simulink model "simulation01"  (R2024a)
settings: Solver=VariableStepAuto  StartTime=0.0  StopTime=50  RelTol=1e-3
values from neighbouring files (symbols this model uses):
  Ax = 0.3    [StateSpace.m]    (also in StateSpace00.m)
  Ay = 0.2    [StateSpace.m]    (also in StateSpace00.m)
  Az = 0.1    [StateSpace.m]    (also in StateSpace00.m)
  Cd = 0.4    [StateSpace.m]    (also in StateSpace00.m)
  g = 9.81    [StateSpace.m]    (also in StateSpace00.m = 9.8)
  Ix = (1/12) * m * (b^2 + c^2)    (= 0.416666666667)    [StateSpace.m]    (also in StateSpace00.m = 10)
  Iy = (1/12) * m * (a^2 + c^2)    (= 0.683333333333)    [StateSpace.m]    (also in StateSpace00.m = 20)
  Iz = (1/12) * m * (a^2 + b^2)    (= 0.566666666667)    [StateSpace.m]    (also in StateSpace00.m = 30)
  L = 5    [StateSpace.m]
  m = 5    [StateSpace.m]    (also in StateSpace00.m)
  rho = 1.225    [StateSpace.m]    (also in StateSpace00.m)
settings Model: Creator=swh  LastModifiedBy=swh
settings DebuggingCC: UnderSpecifiedDimensionMsg=warning

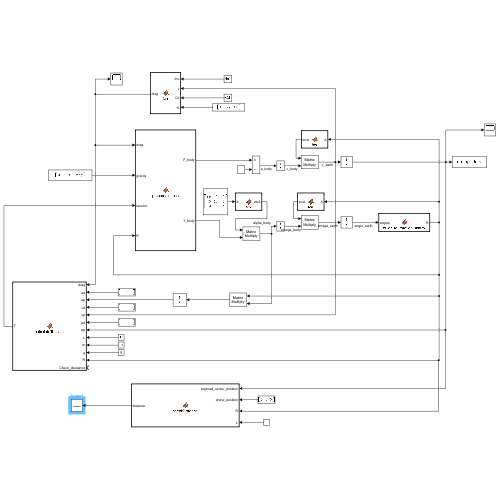
[thumbnail: Simulink's stored preview of the top-level diagram]
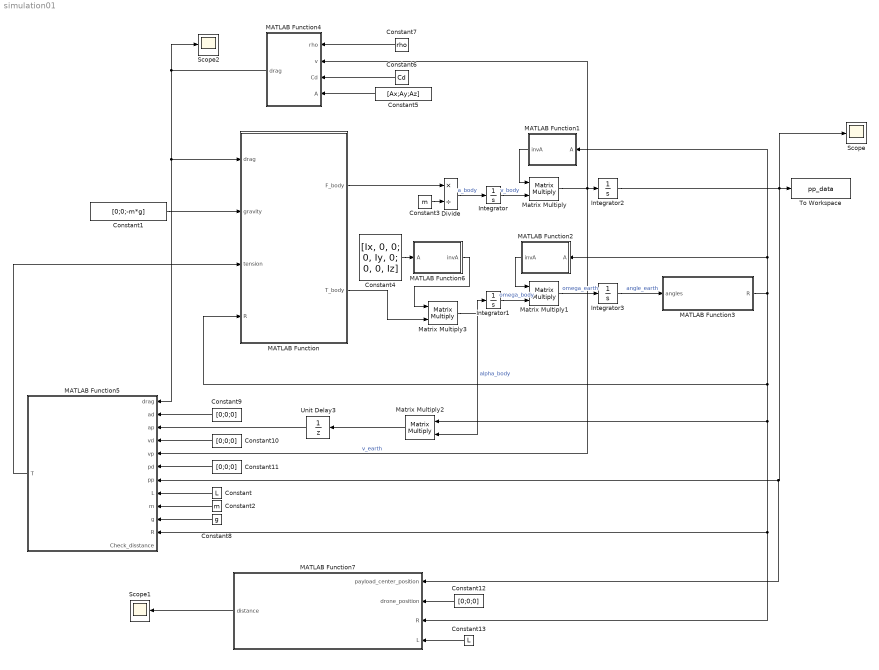
== system simulation01 ==
  Constant : Constant  Value=L
  Constant1 : Constant  Value=[0;0;-m*g]
  Constant{9..12} (4 alike) : Constant  Value=[0;0;0]
  Constant13 : Constant  Value=L
  Constant2 : Constant  Value=m
  Constant3 : Constant  Value=m
  Constant4 : Constant  Value=[Ix, 0, 0; 0, Iy, 0; 0, 0, Iz]
  Constant5 : Constant  Value=[Ax;Ay;Az]
  Constant6 : Constant  Value=Cd
  Constant7 : Constant  Value=rho
  Constant8 : Constant  Value=g
  Divide : Product  Inputs=*/
  Integrator : Integrator
  Integrator1 : Integrator
  Integrator2 : Integrator  InitialCondition=[0,-3,-4]
  Integrator3 : Integrator
  MATLAB Function : MATLAB Function  TreatAsAtomicUnit=on
  MATLAB Function1 : MATLAB Function  TreatAsAtomicUnit=on
  MATLAB Function2 : MATLAB Function  TreatAsAtomicUnit=on
  MATLAB Function3 : MATLAB Function  TreatAsAtomicUnit=on
  MATLAB Function4 : MATLAB Function  TreatAsAtomicUnit=on
  MATLAB Function5 : MATLAB Function  TreatAsAtomicUnit=on
  MATLAB Function6 : MATLAB Function  TreatAsAtomicUnit=on
  MATLAB Function7 : MATLAB Function  TreatAsAtomicUnit=on
  Matrix Multiply{,1..3} (4 alike) : Product  Multiplication=Matrix(*)
  Scope : Scope
  Scope1 : Scope
  Scope2 : Scope
  To Workspace : ToWorkspace  VariableName=pp_data  SaveFormat=Structure With Time  SampleTime=-1
  Unit Delay3 : UnitDelay  SampleTime=-1  HasFrameUpgradeWarning=on
  wires:
  Constant1/1 -> MATLAB Function/2(gravity)
  MATLAB Function/1(F_body) -> Divide/1
  Constant3/1 -> Divide/2
  MATLAB Function/2(T_body) -> Matrix Multiply3/2
  Divide/1 -> Integrator/1  "a_body"
  Matrix Multiply3/1 -> Matrix Multiply2/2, Integrator1/1  "alpha_body"
  Matrix Multiply/1 -> MATLAB Function4/2(v), MATLAB Function5/5(vp), Integrator2/1  "v_earth"
  Matrix Multiply1/1 -> Integrator3/1  "omega_earth"
  Integrator3/1 -> MATLAB Function3/1(angles)  "angle_earth"
  Constant5/1 -> MATLAB Function4/4(A)
  Constant6/1 -> MATLAB Function4/3(Cd)
  Constant7/1 -> MATLAB Function4/1(rho)
  Matrix Multiply2/1 -> Unit Delay3/1
  MATLAB Function4/1(drag) -> MATLAB Function/1(drag), MATLAB Function5/1(drag), Scope2/1
  Constant9/1 -> MATLAB Function5/2(ad)
  Constant10/1 -> MATLAB Function5/4(vd)
  Constant11/1 -> MATLAB Function5/6(pd)
  Constant/1 -> MATLAB Function5/8(L)
  Constant2/1 -> MATLAB Function5/9(m)
  Constant8/1 -> MATLAB Function5/10(g)
  MATLAB Function5/1(T) -> MATLAB Function/3(tension)
  Integrator/1 -> Matrix Multiply/2  "v_body"
  MATLAB Function1/1(invA) -> Matrix Multiply/1
  Integrator1/1 -> Matrix Multiply1/2  "omega_body"
  MATLAB Function2/1(invA) -> Matrix Multiply1/1
  Constant4/1 -> MATLAB Function6/1(A)
  MATLAB Function6/1(invA) -> Matrix Multiply3/1
  MATLAB Function3/1(R) -> MATLAB Function7/3(R), MATLAB Function5/11(R), Matrix Multiply2/1, MATLAB Function/4(R), MATLAB Function2/1(A), MATLAB Function1/1(A)
  Unit Delay3/1 -> MATLAB Function5/3(ap)
  Constant12/1 -> MATLAB Function7/2(drone_position)
  Constant13/1 -> MATLAB Function7/4(L)
  MATLAB Function7/1(distance) -> Scope1/1
  Integrator2/1 -> Scope/1, MATLAB Function7/1(payload_center_position), MATLAB Function5/7(pp), To Workspace/1

== matlab function simulation01/MATLAB Function1 ==
  data: A input; invA output
function invA = fcn(A)
% 计算矩阵 A 的逆
% 输入: A (3x3 矩阵)
% 输出: invA (A 的逆矩阵)
invA = inv(A);  % 使用 MATLAB 的 inv 函数
end

== matlab function simulation01/MATLAB Function ==
  data: drag input size=[3,1]; F_body output size=[3,1]; gravity input size=[3,1]; tension input size=[3,1]; R input size=[3,3]; T_body output size=[3,1]
function [F_body, T_body] = process_forces(drag, gravity, tension, R)
   
    c = 0.8; % The length of the rectangular prism along the z-axis
    r_top = [0;0;0.5 * c];
    % Convert forces from the Earth coordinate system to the body coordinate system
    drag_body = R * drag;
    gravity_body = R * gravity;
    tension_body = R * tension;
    
    % Calculate the resultant force in the body coordinate system
    F_body = drag_body + gravity_body + tension_body;
    
    % In this example, assume the torque is zero (this can be adjusted based on specific requirements)
    p_top = R * r_top;
    r = - p_top;
    T_body = cross(r, tension);  % Calculate the torque based on actual needs
    
end

== matlab function simulation01/MATLAB Function2 ==
  data: A input; invA output
function invA = fcn(A)
% 计算矩阵 A 的逆
% 输入: A (3x3 矩阵)
% 输出: invA (A 的逆矩阵)
invA = inv(A);  % 使用 MATLAB 的 inv 函数
end

== matlab function simulation01/MATLAB Function3 ==
  data: angles input; R output
function R = euler_to_rotation_matrix(angles)
% Calculate the rotation matrix for the given Euler angles
% Input: angles (3x1 column vector) containing Euler angles [phi; theta; psi]
% Output: R (3x3 rotation matrix)

% Extract Euler angles
phi = angles(1);   % Angle around the x-axis
theta = angles(2); % Angle around the y-axis
psi = angles(3);   % Angle around the z-axis

% Rotation matrix around the x-axis
Rx = [1, 0, 0;
      0, cos(phi), -sin(phi);
      0, sin(phi), cos(phi)];

% Rotation matrix around the y-axis
Ry = [cos(theta), 0, sin(theta);
      0, 1, 0;
      -sin(theta), 0, cos(theta)];

% Rotation matrix around the z-axis
Rz = [cos(psi), -sin(psi), 0;
      sin(psi), cos(psi), 0;
      0, 0, 1];

% Calculate the final rotation matrix
R = Rz * Ry * Rx;
end

== matlab function simulation01/MATLAB Function4 ==
  data: rho input; drag output size=[3,1]; v input size=[3,1]; Cd input; A input
function drag = fcn(rho, v, Cd, A)
    % 计算速度的大小
    speed = sqrt(v(1)^2 + v(2)^2 + v(3)^2);
    
    % 计算速度方向向量（单位向量）
    if speed ~= 0
        unit_v = v / speed;
    else
        % 如果速度为零，单位向量也为零
        unit_v = [0; 0; 0];
    end
    
    % 计算拖拽力的大小
    drag_magnitude = 0.5 * rho * speed^2 * Cd * A;
    
    % 计算拖拽力的方向和大小
    drag = -drag_magnitude .* unit_v; % 按元素相乘

end

== matlab function simulation01/MATLAB Function5 ==
  data: drag input; ad input; T output size=[3,1]; ap input; vd input; vp input; pd input; pp input; L input; m input; g input; R input; Check_disstance input
function T = calculateTension(drag, ad, ap, vd, vp, pd, pp, L, m, g, R, Check_disstance)
% Calculate the components of the rope tension in the x, y, and z directions for a 3D pendulum
%
% Inputs:
%   ad, ap - Acceleration components of the object at two different points
%   vd, vp - Velocity components of the object at two different points
%   pd, pp - Coordinates of the suspension point and the object
%   L - Length of the rope
%   m - Mass of the object
%   g - Acceleration due to gravity
%
% Output:
%   T - Tension components in the x, y, and z directions, in the form [Tx; Ty; Tz]

% Calculate displacement vector
c = 0.8;
r_top = [0;0;0.5 * c];
p_top = R * r_top;
p_connection = p_top + pp;

ax = ap(1) - ad(1);
ay = ap(2) - ad(2);
az = ap(3) - ad(3);

vx = vp(1) - vd(1);
vy = vp(2) - vd(2);
vz = vp(3) - vd(3);

dx = pd(1) - p_connection(1);
dy = pd(2) - p_connection(2);
dz = pd(3) - p_connection(3);

% Calculate unit vector
T_unit = [dx; dy; dz] / L;

% Calculate the magnitude of velocity
v = sqrt(vx^2 + vy^2 + vz^2);

% Calculate centripetal acceleration
a_c = v^2 / L;

% Calculate gravitational force component
F_g = -m * g;

% Calculate external force components

F_x = drag(1);
F_y = drag(2);
F_z = drag(3);


% Calculate fictitious force
ff_x =  - m * ad(1);
ff_y =  - m * ad(2);
ff_z =  - m * ad(3);

% Calculate tension magnitude

T_magnitude = ( -(F_x + ff_x) * dx  -(F_y + ff_y)  * dy  -(F_z + ff_z) * dz - F_g * dz) / L + m * a_c / L;

% Calculate the tension components in the x, y, and z directions


T = T_magnitude * T_unit;

% Output the tension components in the x, y, and z directions
end

== matlab function simulation01/MATLAB Function6 ==
  data: A input; invA output
function invA = fcn(A)
% 计算矩阵 A 的逆
% 输入: A (3x3 矩阵)
% 输出: invA (A 的逆矩阵)
invA = inv(A);  % 使用 MATLAB 的 inv 函数
end

== matlab function simulation01/MATLAB Function7 ==
  data: payload_center_position input size=[3,1]; drone_position input size=[3,1]; R input size=[3,3]; distance output; L input
function distance = checkDistance(payload_center_position, drone_position, R, L)
    % payload_center_position: 负载中心位置，格式为 [x1, y1, z1]
    % drone_position: 无人机位置，格式为 [x2, y2, z2]
    % R: 旋转矩阵
    % L: 给定的长度阈值（在当前版本中未使用）

    % 定义绳索连接点相对于负载中心的位置（局部坐标系）
    r_top = [0; 0; 0.4];
    
    % 计算绳索连接点在全局坐标系中的位置
    p_top = R * r_top;
    connection_position = payload_center_position + p_top;
    
    % 计算无人机位置和绳索连接点之间的欧几里得距离
    distance = norm(drone_position - connection_position);
end
